simulink model "Modelo_global_NL_sin_LC_NL"  (R2023a)
settings: Solver=VariableStepAuto  StartTime=0.0  StopTime=1  MaxStep=1e-4  RelTol=1e-3
undefined symbols (not defined in the file or in its folder): alpha_Cu, b_eq, Cts, J_eq, k_l, lambda, Ld, Lls, Lq, Pp, r, Rs_ref, Rts, Ts_ref
libraries: SignalEditorBlockLib x3
settings Model: Creator=Renzo  LastModifiedBy=tobip
settings DataIOCC: ExternalInput=T_amb
settings DebuggingCC: UnderSpecifiedDimensionMsg=warning

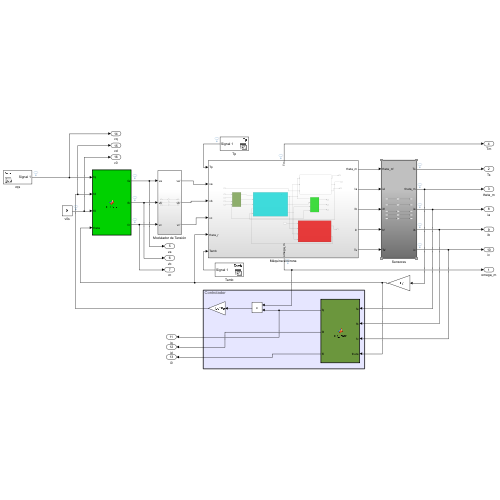
[thumbnail: Simulink's stored preview of the top-level diagram]
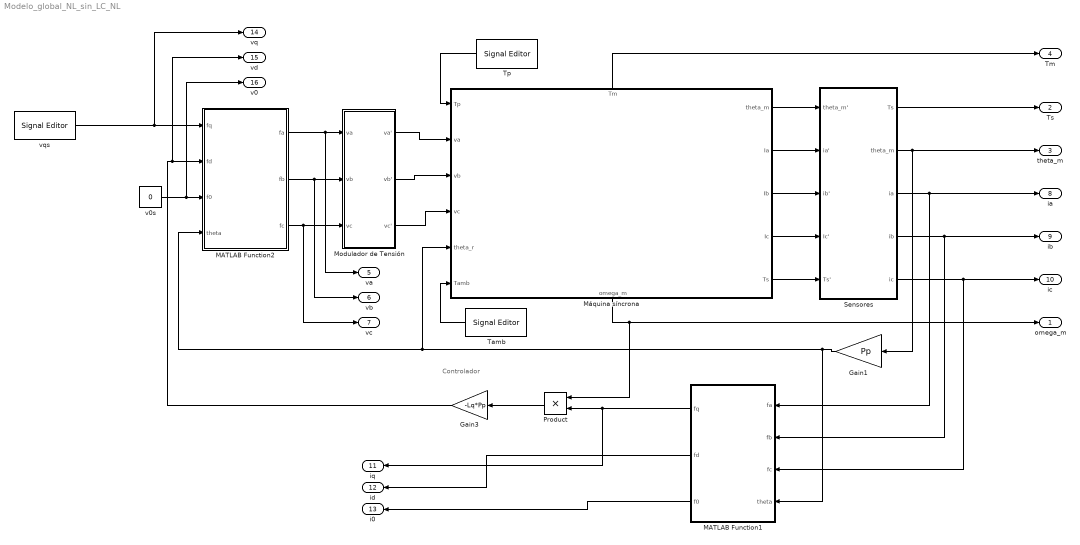
== system Modelo_global_NL_sin_LC_NL ==
  note: Controlador
  Gain1 : Gain  Gain=Pp
  Gain3 : Gain  Gain=-Lq*Pp
  MATLAB Function1 : MATLAB Function  TreatAsAtomicUnit=on
  MATLAB Function2 : MATLAB Function  TreatAsAtomicUnit=on
  Modulador de Tensión : Subsystem
  Máquina síncrona : Subsystem
      settings: PortSchema="{\"entries\":[{\"content\":{\"sides\":[{\"content\":{\"connectorIds\":[\"In1\",\"In2\",\"In3\",\"In4\",\"In5\",\"In6\"]},\"type\":\"ConnectorPlacement.EquallySpacedRectSide\",\"uuid\":\"548fbf6f-bb54-461c-a3ca-ae13566b19bb\"},{\"content\":{\"connectorIds\":[\"Out1\",\"Out2\",\"Out3\",\"Out4\",\"Out5\"],\"side\":\"RIGHT\"},\"type\":\"ConnectorPlacement.EquallySpacedRectSide\",\"uuid\":\"c9a1420a-e64d-4e02-ad2b-140f5c663a2c\"},{\"content\":{\"connectorIds\":[\"Out7\"],\"side\":\"TOP\"},\"type\":\"ConnectorPlacement.EquallySpacedRectSide\",\"uuid\":\"df4aae34-4e90-4058-9a3e-cb814e1189cf\"},{\"content\":{\"connectorIds\":[\"Out6\"],\"side\":\"BOTTOM\"},\"type\":\"ConnectorPlacement.EquallySpacedRectSide\",\"uuid\":\"ddc2a780-dbd9-4ee7-a70a-9225aa3ce731\"}]},\"type\":\"ConnectorPlacement.EquallySpacedConnector\",\"uuid\":\"8e0529f1-5fe4-4179-9319-aba0984f7167\"}],\"packageUris\":[\"http://schema.mathworks.com/mf0/Connector/R2020b\"],\"version\":\"1.0\"}"
  Product : Product
  Sensores : Subsystem
  Tamb : SignalEditorBlockLib/Signal Editor  FileName=senal_Tamb.mat  ActiveScenario=Tamb  ActiveSignal=Constant  IsBus=off  OutputBusObjectStr=Bus: BusObject  SampleTime=0  Interpolate=off  ZeroCross=off  OutputAfterFinalValue=Setting to zero  Unit=inherit  PreserveSignalName=on  ApplySigPropsToAllScenarios=on
  Tp : SignalEditorBlockLib/Signal Editor  FileName=senal_Tp.mat  ActiveScenario=Tp  ActiveSignal=Pulse  IsBus=off  OutputBusObjectStr=Bus: BusObject  SampleTime=0  Interpolate=off  ZeroCross=off  OutputAfterFinalValue=Setting to zero  Unit=inherit  PreserveSignalName=on  ApplySigPropsToAllScenarios=off
  v0s : Constant  Value=0
  vqs : SignalEditorBlockLib/Signal Editor  FileName=senal_vqs.mat  ActiveScenario=Vqs  ActiveSignal=Pulse  IsBus=off  OutputBusObjectStr=Bus: BusObject  SampleTime=0  Interpolate=off  ZeroCross=off  OutputAfterFinalValue=Setting to zero  Unit=inherit  PreserveSignalName=on  ApplySigPropsToAllScenarios=on
  omega_m : Outport
  Ts : Outport  Port=2
  theta_m : Outport  Port=3
  Tm : Outport  Port=4
  va : Outport  Port=5
  vb : Outport  Port=6
  vc : Outport  Port=7
  ia : Outport  Port=8
  ib : Outport  Port=9
  ic : Outport  Port=10
  iq : Outport  Port=11
  id : Outport  Port=12
  i0 : Outport  Port=13
  vq : Outport  Port=14
  vd : Outport  Port=15
  v0 : Outport  Port=16
  wires:
  Máquina síncrona/3(Ib) -> Sensores/3(ib')
  Máquina síncrona/5(Ts) -> Sensores/5(Ts')
  Máquina síncrona/4(Ic) -> Sensores/4(Ic')
  Sensores/1(Ts) -> Ts/1
  Sensores/2(theta_m) -> theta_m/1, Gain1/1
  Máquina síncrona/2(Ia) -> Sensores/2(ia')
  Máquina síncrona/1(theta_m) -> Sensores/1(theta_m')
  MATLAB Function2/1(fa) -> va/1, Modulador de Tensión/1(va)
  MATLAB Function2/2(fb) -> vb/1, Modulador de Tensión/2(vb)
  MATLAB Function2/3(fc) -> Modulador de Tensión/3(vc), vc/1
  Modulador de Tensión/1(va') -> Máquina síncrona/2(va)
  Modulador de Tensión/2(vb') -> Máquina síncrona/3(vb)
  Modulador de Tensión/3(vc') -> Máquina síncrona/4(vc)
  vqs/1 -> MATLAB Function2/1(fq), vq/1
  v0s/1 -> MATLAB Function2/3(f0), v0/1
  Máquina síncrona/7(Tm) -> Tm/1
  Tp/1 -> Máquina síncrona/1(Tp)
  Tamb/1 -> Máquina síncrona/6(Tamb)
  Gain3/1 -> MATLAB Function2/2(fd), vd/1
  MATLAB Function1/1(fq) -> iq/1, Product/2
  MATLAB Function1/2(fd) -> id/1
  MATLAB Function1/3(f0) -> i0/1
  Gain1/1 -> MATLAB Function1/4(theta), Máquina síncrona/5(theta_r), MATLAB Function2/4(theta)
  Sensores/3(ia) -> MATLAB Function1/1(fa), ia/1
  Máquina síncrona/6(omega_m) -> omega_m/1, Product/1
  Sensores/5(ic) -> MATLAB Function1/3(fc), ic/1
  Sensores/4(ib) -> MATLAB Function1/2(fb), ib/1
  Product/1 -> Gain3/1

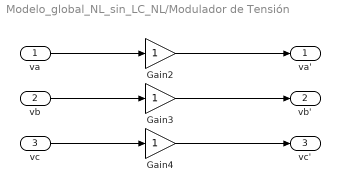
== system Modelo_global_NL_sin_LC_NL/Modulador de Tensión ==
  va : Inport
  vb : Inport  Port=2
  vc : Inport  Port=3
  Gain2 : Gain
  Gain3 : Gain
  Gain4 : Gain
  va' : Outport
  vb' : Outport  Port=2
  vc' : Outport  Port=3
  wires:
  vb/1 -> Gain3/1
  Gain4/1 -> vc'/1
  Gain2/1 -> va'/1
  va/1 -> Gain2/1
  vc/1 -> Gain4/1
  Gain3/1 -> vb'/1

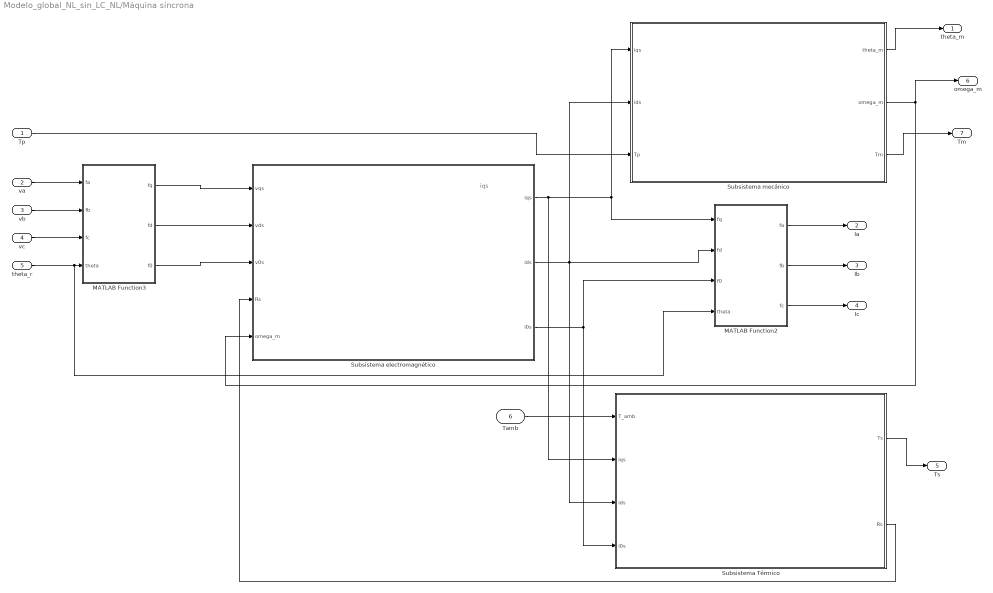
== system Modelo_global_NL_sin_LC_NL/Máquina síncrona ==
  note: iqs
  Tp : Inport
  va : Inport  Port=2
  vb : Inport  Port=3
  vc : Inport  Port=4
  theta_r : Inport  Port=5
  Tamb : Inport  Port=6
  MATLAB Function2 : MATLAB Function  TreatAsAtomicUnit=on
  MATLAB Function3 : MATLAB Function  TreatAsAtomicUnit=on
  Subsistema Térmico : Subsystem
  Subsistema electromagnético : Subsystem
  Subsistema mecánico : Subsystem
  theta_m : Outport
  Ia : Outport  Port=2
  Ib : Outport  Port=3
  Ic : Outport  Port=4
  Ts : Outport  Port=5
  omega_m : Outport  Port=6
  Tm : Outport  Port=7
  wires:
  MATLAB Function3/1(fq) -> Subsistema electromagnético/1(vqs)
  Subsistema electromagnético/1(iqs) -> Subsistema Térmico/2(iqs), Subsistema mecánico/1(iqs), MATLAB Function2/1(fq)
  Subsistema electromagnético/2(ids) -> MATLAB Function2/2(fd), Subsistema Térmico/3(ids), Subsistema mecánico/2(ids)
  Subsistema mecánico/2(omega_m) -> omega_m/1, Subsistema electromagnético/5(omega_m)
  MATLAB Function3/3(f0) -> Subsistema electromagnético/3(v0s)
  Subsistema electromagnético/3(i0s) -> MATLAB Function2/3(f0), Subsistema Térmico/4(i0s)
  Subsistema mecánico/1(theta_m) -> theta_m/1
  Subsistema Térmico/2(Rs) -> Subsistema electromagnético/4(Rs)
  MATLAB Function2/3(fc) -> Ic/1
  MATLAB Function3/2(fd) -> Subsistema electromagnético/2(vds)
  MATLAB Function2/2(fb) -> Ib/1
  Tp/1 -> Subsistema mecánico/3(Tp)
  va/1 -> MATLAB Function3/1(fa)
  vc/1 -> MATLAB Function3/3(fc)
  theta_r/1 -> MATLAB Function2/4(theta), MATLAB Function3/4(theta)
  vb/1 -> MATLAB Function3/2(fb)
  Subsistema Térmico/1(Ts) -> Ts/1
  Tamb/1 -> Subsistema Térmico/1(T_amb)
  MATLAB Function2/1(fa) -> Ia/1
  Subsistema mecánico/3(Tm) -> Tm/1

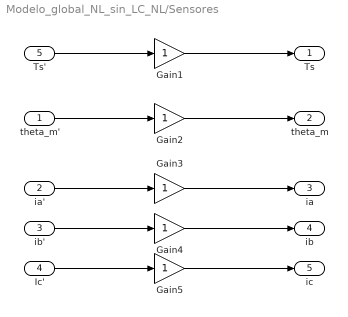
== system Modelo_global_NL_sin_LC_NL/Sensores ==
  theta_m' : Inport
  ia' : Inport  Port=2
  ib' : Inport  Port=3
  Ic' : Inport  Port=4
  Ts' : Inport  Port=5
  Gain{1..5} (5 alike) : Gain
  Ts : Outport
  theta_m : Outport  Port=2
  ia : Outport  Port=3
  ib : Outport  Port=4
  ic : Outport  Port=5
  wires:
  Gain1/1 -> Ts/1
  Ic'/1 -> Gain5/1
  Gain4/1 -> ib/1
  ib'/1 -> Gain4/1
  Gain5/1 -> ic/1
  ia'/1 -> Gain3/1
  theta_m'/1 -> Gain2/1
  Ts'/1 -> Gain1/1
  Gain3/1 -> ia/1
  Gain2/1 -> theta_m/1

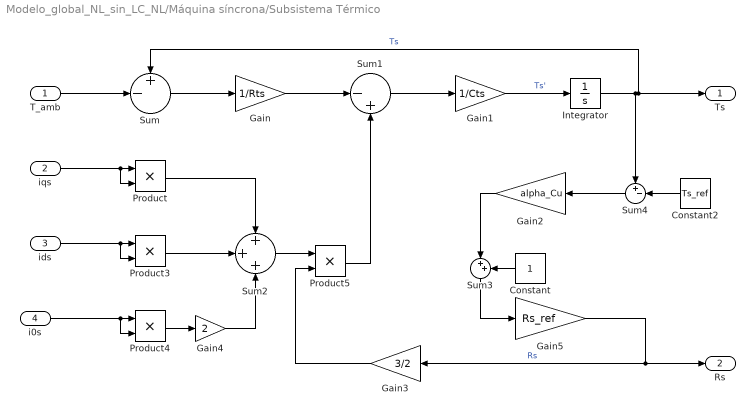
== system Modelo_global_NL_sin_LC_NL/Máquina síncrona/Subsistema Térmico ==
  T_amb : Inport
  iqs : Inport  Port=2
  ids : Inport  Port=3
  i0s : Inport  Port=4
  Constant : Constant
  Constant2 : Constant  Value=Ts_ref
  Gain : Gain  Gain=1/Rts
  Gain1 : Gain  Gain=1/Cts
  Gain2 : Gain  Gain=alpha_Cu
  Gain3 : Gain  Gain=3/2
  Gain4 : Gain  Gain=2
  Gain5 : Gain  Gain=Rs_ref
  Integrator : Integrator
  Product{,3..5} (4 alike) : Product
  Sum : Sum  Inputs=+-|
  Sum1 : Sum  Inputs=|-+
  Sum2 : Sum  Inputs=+++
  Sum3 : Sum  Inputs=|++
  Sum4 : Sum  Inputs=+-|
  Ts : Outport
  Rs : Outport  Port=2
  wires:
  Gain/1 -> Sum1/1
  iqs/1 -> Product/2, Product/1
  ids/1 -> Product3/2, Product3/1
  Integrator/1 -> Ts/1, Sum/1, Sum4/1  "Ts"
  Constant/1 -> Sum3/2
  Product3/1 -> Sum2/2
  Product5/1 -> Sum1/2
  Sum/1 -> Gain/1
  i0s/1 -> Product4/2, Product4/1
  Gain1/1 -> Integrator/1  "Ts'"
  Sum4/1 -> Gain2/1
  Constant2/1 -> Sum4/2
  Sum1/1 -> Gain1/1
  Product4/1 -> Gain4/1
  Sum2/1 -> Product5/1
  Gain2/1 -> Sum3/1
  Product/1 -> Sum2/1
  T_amb/1 -> Sum/2
  Gain3/1 -> Product5/2
  Gain4/1 -> Sum2/3
  Sum3/1 -> Gain5/1
  Gain5/1 -> Gain3/1, Rs/1  "Rs"

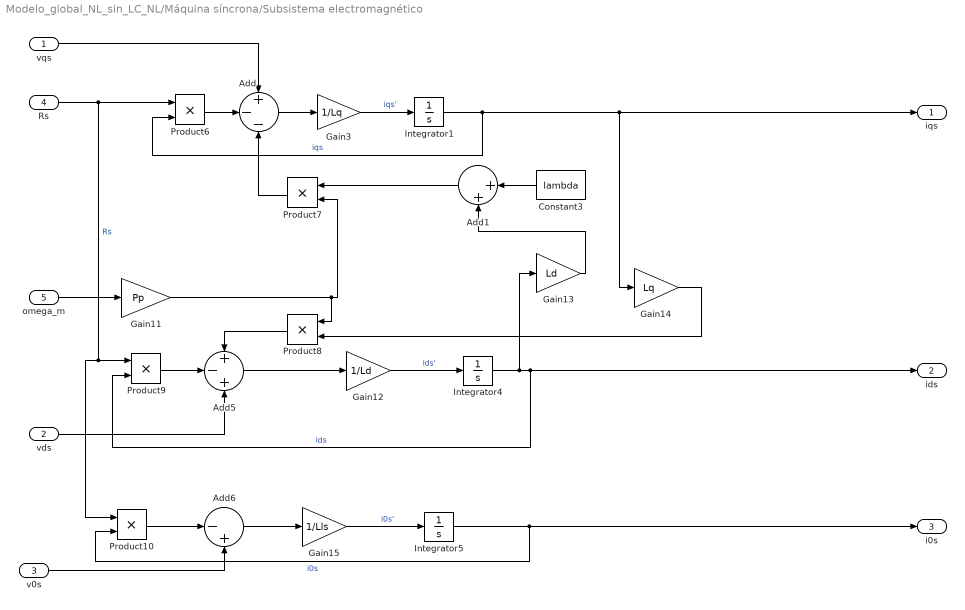
== system Modelo_global_NL_sin_LC_NL/Máquina síncrona/Subsistema electromagnético ==
  vqs : Inport
  vds : Inport  Port=2
  v0s : Inport  Port=3
  Rs : Inport  Port=4
  omega_m : Inport  Port=5
  Add : Sum  Inputs=+--
  Add1 : Sum  Inputs=|++
  Add5 : Sum  Inputs=+-+
  Add6 : Sum  Inputs=|-+
  Constant3 : Constant  Value=lambda
  Gain11 : Gain  Gain=Pp
  Gain12 : Gain  Gain=1/Ld
  Gain13 : Gain  Gain=Ld
  Gain14 : Gain  Gain=Lq
  Gain15 : Gain  Gain=1/Lls
  Gain3 : Gain  Gain=1/Lq
  Integrator1 : Integrator
  Integrator4 : Integrator
  Integrator5 : Integrator
  Product{6..10} (5 alike) : Product
  iqs : Outport
  ids : Outport  Port=2
  i0s : Outport  Port=3
  wires:
  Add6/1 -> Gain15/1
  vds/1 -> Add5/3
  Gain13/1 -> Add1/2
  Rs/1 -> Product6/1, Product10/1, Product9/1  "Rs"
  Gain14/1 -> Product8/2
  Gain15/1 -> Integrator5/1  "i0s'"
  Add/1 -> Gain3/1
  v0s/1 -> Add6/2
  Integrator1/1 -> Product6/2, Gain14/1, iqs/1  "iqs"
  Gain12/1 -> Integrator4/1  "ids'"
  Gain3/1 -> Integrator1/1  "iqs'"
  Gain11/1 -> Product8/1, Product7/2
  Add5/1 -> Gain12/1
  Integrator5/1 -> i0s/1, Product10/2  "i0s"
  Product9/1 -> Add5/2
  Constant3/1 -> Add1/1
  Product10/1 -> Add6/1
  Product7/1 -> Add/3
  Product8/1 -> Add5/1
  Integrator4/1 -> ids/1, Product9/2, Gain13/1  "ids"
  Add1/1 -> Product7/1
  vqs/1 -> Add/1
  Product6/1 -> Add/2
  omega_m/1 -> Gain11/1

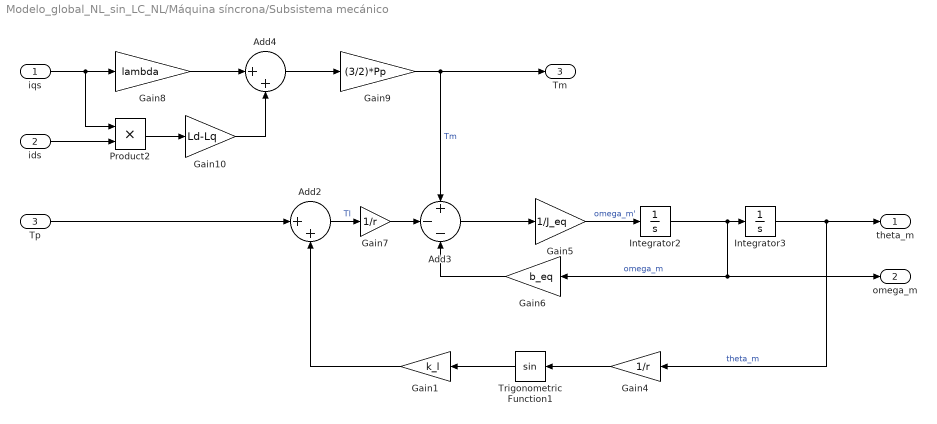
== system Modelo_global_NL_sin_LC_NL/Máquina síncrona/Subsistema mecánico ==
  iqs : Inport
  ids : Inport  Port=2
  Tp : Inport  Port=3
  Add2 : Sum  Inputs=|++
  Add3 : Sum  Inputs=+--
  Add4 : Sum  Inputs=|++
  Gain1 : Gain  Gain=k_l
  Gain10 : Gain  Gain=Ld-Lq
  Gain4 : Gain  Gain=1/r
  Gain5 : Gain  Gain=1/J_eq
  Gain6 : Gain  Gain=b_eq
  Gain7 : Gain  Gain=1/r
  Gain8 : Gain  Gain=lambda
  Gain9 : Gain  Gain=(3/2)*Pp
  Integrator2 : Integrator
  Integrator3 : Integrator
  Product2 : Product
  Trigonometric Function1 : Trigonometry
  theta_m : Outport
  omega_m : Outport  Port=2
  Tm : Outport  Port=3
  wires:
  Gain4/1 -> Trigonometric Function1/1
  Integrator2/1 -> omega_m/1, Gain6/1, Integrator3/1  "omega_m"
  iqs/1 -> Product2/1, Gain8/1
  Gain6/1 -> Add3/3
  Gain9/1 -> Tm/1, Add3/1  "Tm"
  Gain8/1 -> Add4/1
  Gain5/1 -> Integrator2/1  "omega_m'"
  Add2/1 -> Gain7/1  "Tl"
  Integrator3/1 -> theta_m/1, Gain4/1  "theta_m"
  Add4/1 -> Gain9/1
  Product2/1 -> Gain10/1
  Gain7/1 -> Add3/2
  Add3/1 -> Gain5/1
  Gain10/1 -> Add4/2
  Tp/1 -> Add2/1
  ids/1 -> Product2/2
  Trigonometric Function1/1 -> Gain1/1
  Gain1/1 -> Add2/2

== matlab function Modelo_global_NL_sin_LC_NL/Máquina síncrona/MATLAB Function2 ==
  data: fq input; fa output size=1; fd input; f0 input; theta input; fb output size=1; fc output size=1
function [fa,fb,fc] = TI_Park(fq,fd,f0,theta)

f = [     cos(theta)              sin(theta)         1;
       cos(theta - (2*pi)/3)   sin(theta - (2*pi)/3)   1;
       cos(theta + (2*pi)/3)   sin(theta + (2*pi)/3)   1];

resultados = f*[fq;fd;f0];
fa = resultados(1);
fb = resultados(2);
fc = resultados(3);

== matlab function Modelo_global_NL_sin_LC_NL/Máquina síncrona/MATLAB Function3 ==
  data: fa input; fq output size=1; fb input; fc input; theta input; fd output size=1; f0 output size=1
function [fq,fd,f0] = TD_Park(fa,fb,fc,theta)

f = (2/3)*[cos(theta)  cos(theta - (2*pi)/3)   cos(theta + (2*pi)/3);
           sin(theta)  sin(theta - (2*pi)/3)   sin(theta + (2*pi)/3);
              1/2              1/2                     1/2         ];

resultados = f*[fa;fb;fc];
fq = resultados(1);
fd = resultados(2);
f0 = resultados(3);

== matlab function Modelo_global_NL_sin_LC_NL/MATLAB Function1 ==
  data: fa input; fq output size=1; fb input; fc input; theta input; fd output size=1; f0 output size=1
function [fq,fd,f0] = TD_Park(fa,fb,fc,theta)

f = (2/3)*[cos(theta)  cos(theta - (2*pi)/3)   cos(theta + (2*pi)/3);
           sin(theta)  sin(theta - (2*pi)/3)   sin(theta + (2*pi)/3);
              1/2              1/2                     1/2         ];

resultados = f*[fa;fb;fc];
fq = resultados(1);
fd = resultados(2);
f0 = resultados(3);

== matlab function Modelo_global_NL_sin_LC_NL/MATLAB Function2 ==
  data: fq input; fa output size=1; fd input; f0 input; theta input; fb output size=1; fc output size=1
function [fa,fb,fc] = TI_Park(fq,fd,f0,theta)

f = [     cos(theta)              sin(theta)         1;
       cos(theta - (2*pi)/3)   sin(theta - (2*pi)/3)   1;
       cos(theta + (2*pi)/3)   sin(theta + (2*pi)/3)   1];

resultados = f*[fq;fd;f0];
fa = resultados(1);
fb = resultados(2);
fc = resultados(3);
